simulink model "lab"  (R2024b)
settings: Solver=VariableStepAuto  StartTime=0.0  StopTime=10.0  MaxStep=1  RelTol=1e-3
values from neighbouring files (symbols this model uses):
  c_p = 1000    [Copy_2_of_Lab_433.m]    (also in Copy_of_Lab_433.m; Lab_433.m)
  C_vp = c_p*p_p*V_wp    (= 75000)    [Copy_2_of_Lab_433.m]    (also in Copy_of_Lab_433.m; Lab_433.m = 300000)
  C_vw = c_p*p_p*V_we    (= 300000)    [Copy_2_of_Lab_433.m]    (also in Copy_of_Lab_433.m; Lab_433.m = 600000)
  czas_skok = 3000    [Copy_2_of_Lab_433.m]    (also in Copy_of_Lab_433.m = 500; Lab_433.m)
  dPg = 10000    [Copy_2_of_Lab_433.m]    (also in Copy_of_Lab_433.m = 0; Lab_433.m = 2000)
  dTzew = 0    [Copy_2_of_Lab_433.m]    (also in Copy_of_Lab_433.m; Lab_433.m)
  f_pN = 0.01    [Copy_2_of_Lab_433.m]    (also in Copy_of_Lab_433.m; Lab_433.m)
  K_1 = (0.6*P_gN)/(T_wewn-T_zewn)    (= 150)    [Copy_2_of_Lab_433.m]    (also in Copy_of_Lab_433.m; Lab_433.m)
  K_d = (K_p*(T_wewn-T_pn))/(T_pn-T_zewn)    (= 100.571428571)    [Copy_2_of_Lab_433.m]    (also in Copy_of_Lab_433.m; Lab_433.m)
  K_p = (P_gN-K_1*(T_wewn-T_zewn)-c_p*p_p*f_pN*(T_wewn-T_zewn))/(T_wewn-T_pn)    (= 704)    [Copy_2_of_Lab_433.m]    (also in Copy_of_Lab_433.m; Lab_433.m)
  P_gN0 = P_p_Pg(k)    [Copy_2_of_Lab_433.m]    (also in Copy_of_Lab_433.m = 10000; Lab_433.m = 10000)
  p_p = 1.2    [Copy_2_of_Lab_433.m]    (also in Copy_of_Lab_433.m; Lab_433.m)
  T_p0 = (K_p*(T_wewn0)+K_d*T_zewn0)/(K_p+K_d)    (= 15)    [Copy_2_of_Lab_433.m]    (also in Copy_of_Lab_433.m; Lab_433.m)
  T_wewn0 = T_zewn0 + (P_gN0)/(K_1+c_p*p_p*f_pN0+(K_p*K_d)/(K_p+K_d))    (= 20)    [Copy_2_of_Lab_433.m]    (also in Copy_of_Lab_433.m; Lab_433.m)
  T_zewn0 = P_p_T_zew(k)    [Copy_2_of_Lab_433.m]    (also in Copy_of_Lab_433.m = -20; Lab_433.m = -20)
settings Model: Creator=userbrigh  LastModifiedBy=userbrigh

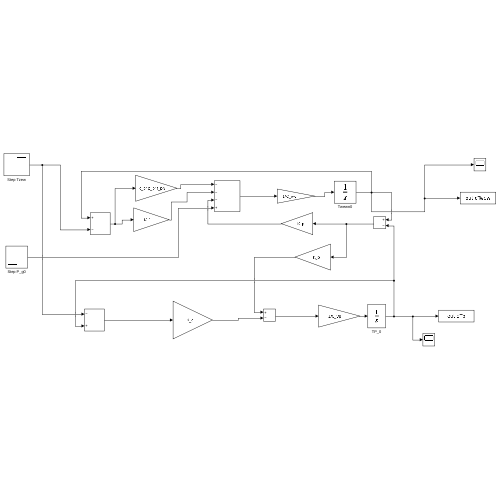
[thumbnail: Simulink's stored preview of the top-level diagram]
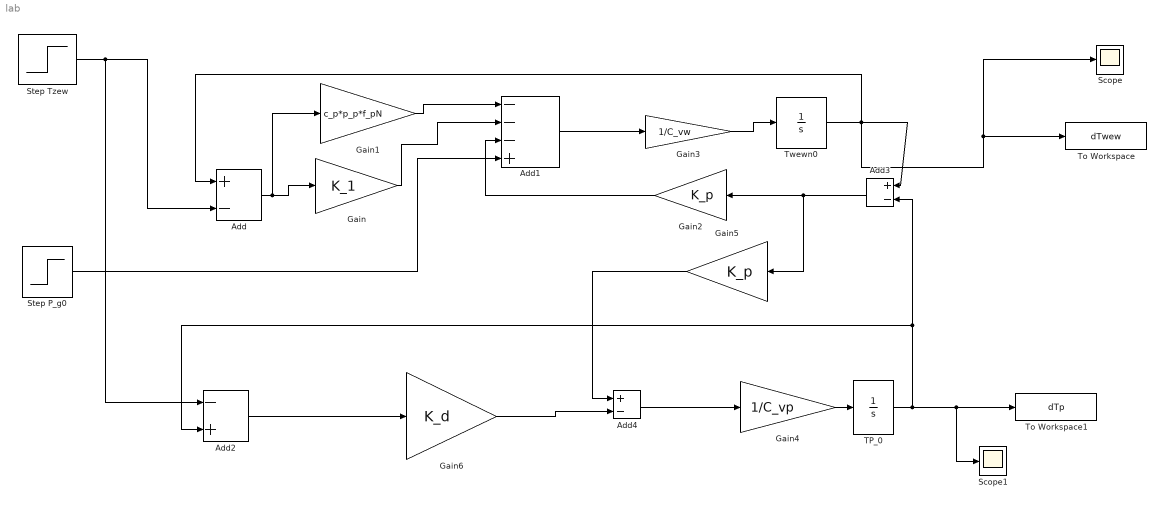
== system lab ==
  Add : Sum  Inputs=+-
  Add1 : Sum  Inputs=---+
  Add2 : Sum  Inputs=-+
  Add3 : Sum  Inputs=+-
  Add4 : Sum  Inputs=+-
  Gain : Gain  Gain=K_1
  Gain1 : Gain  Gain=c_p*p_p*f_pN
  Gain2 : Gain  Gain=K_p
  Gain3 : Gain  Gain=1/C_vw
  Gain4 : Gain  Gain=1/C_vp
  Gain5 : Gain  Gain=K_p
  Gain6 : Gain  Gain=K_d
  Scope : Scope
  Scope1 : Scope
  Step P_g0 : Step  Time=czas_skok  Before=P_gN0  After=P_gN0+dPg  SampleTime=0
  Step Tzew : Step  Time=czas_skok  Before=T_zewn0  After=T_zewn0+dTzew  SampleTime=0
  TP_0 : Integrator  InitialCondition=T_p0
  To Workspace : ToWorkspace  VariableName=dTwew  SampleTime=-1
  To Workspace1 : ToWorkspace  VariableName=dTp  SampleTime=-1
  Twewn0 : Integrator  InitialCondition=T_wewn0
  wires:
  Twewn0/1 -> Scope/1, To Workspace/1, Add/1, Add3/1
  TP_0/1 -> Add2/2, Add3/2, Scope1/1, To Workspace1/1
  Add3/1 -> Gain5/1, Gain2/1
  Step Tzew/1 -> Add2/1, Add/2
  Add/1 -> Gain1/1, Gain/1
  Gain/1 -> Add1/2
  Gain1/1 -> Add1/1
  Add1/1 -> Gain3/1
  Gain2/1 -> Add1/3
  Step P_g0/1 -> Add1/4
  Add2/1 -> Gain6/1
  Gain4/1 -> TP_0/1
  Gain3/1 -> Twewn0/1
  Gain5/1 -> Add4/1
  Gain6/1 -> Add4/2
  Add4/1 -> Gain4/1
